simulink model "Subsystem"  (R2020b)
settings: Solver=FixedStepAuto  StartTime=0.0  StopTime=10.0  FixedStep=0.2  RelTol=1e-3
settings Model: Creator=shubham sharma  LastModifiedBy=shubham sharma
settings DataIOCC: SaveOutput=off  SaveTime=off

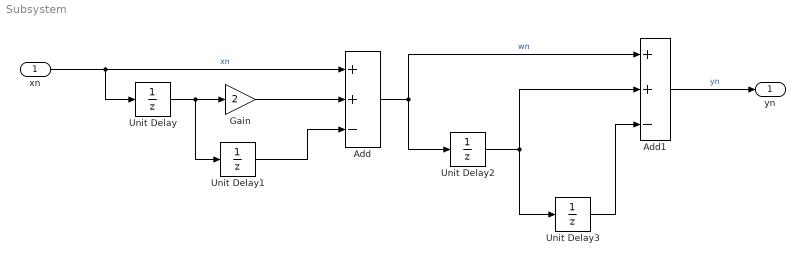
== system Subsystem ==
  xn : Inport  OutDataTypeStr=double  PortDimensions=1
  Add : Sum  Inputs=++-
  Add1 : Sum  Inputs=++-
  Gain : Gain  Gain=2
  Unit Delay{,1..3} (4 alike) : UnitDelay  SampleTime=-1  HasFrameUpgradeWarning=on
  yn : Outport  OutDataTypeStr=double  PortDimensions=1  SampleTime=[0.20000000000000001,0]
  wires:
  Unit Delay2/1 -> Add1/2, Unit Delay3/1
  Unit Delay/1 -> Gain/1, Unit Delay1/1
  Add/1 -> Add1/1, Unit Delay2/1  "wn"
  xn/1 -> Add/1, Unit Delay/1  "xn"
  Unit Delay3/1 -> Add1/3
  Gain/1 -> Add/2
  Unit Delay1/1 -> Add/3
  Add1/1 -> yn/1  "yn"
